simulink model "thermal_analysis"  (R2023b)
settings: Solver=VariableStepAuto  StartTime=0.0  StopTime=10.0  RelTol=1e-3
undefined symbols (not defined in the file): P_diode, P_mosfet, R_case_heatsink, R_heatsink_ambient, R_junction_case_diode, R_junction_case_mosfet, T_ambient
libraries: spsSeriesRLCBranchLib x6, spsControlledCurrentSourceLib x2, spsDCVoltageSourceLib x2, spsVoltageMeasurementLib x2, sps_lib x1
settings Model: Creator=ATAY  LastModifiedBy=ATAY

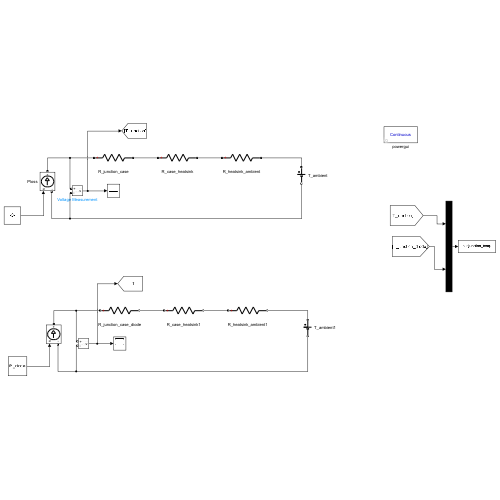
[thumbnail: Simulink's stored preview of the top-level diagram]
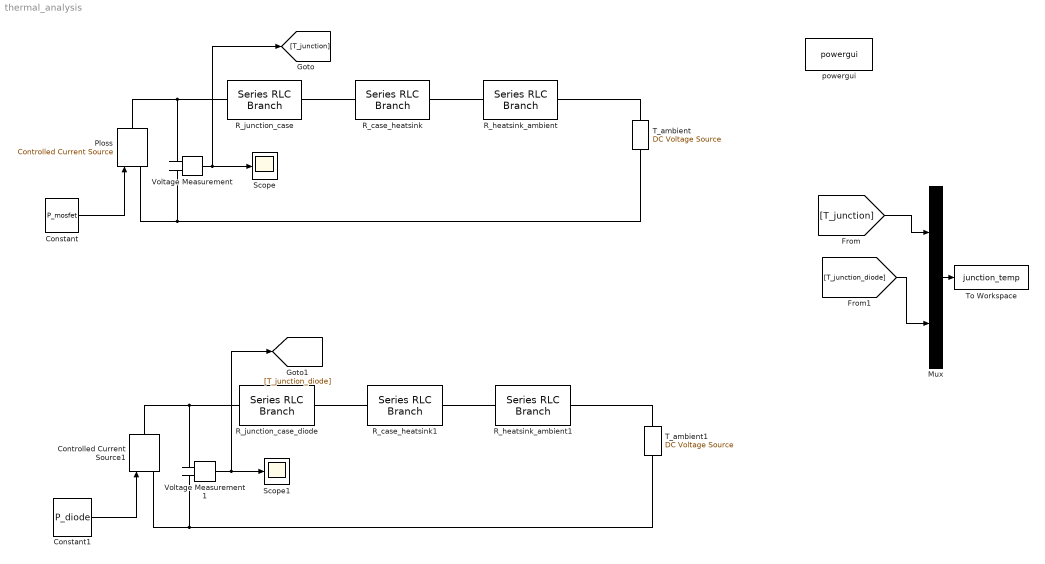
== system thermal_analysis ==
  Constant : Constant  Value=P_mosfet
  Constant1 : Constant  Value=P_diode
  Controlled Current Source1 : spsControlledCurrentSourceLib/Controlled Current Source  Initialize=on  Source_Type=DC  Amplitude=0  Phase=0  Frequency=0  Measurements=None
  Mux : Mux  Inputs=2
  Ploss : spsControlledCurrentSourceLib/Controlled Current Source  Initialize=on  Source_Type=DC  Amplitude=0  Phase=0  Frequency=0  Measurements=None
  R_case_heatsink : spsSeriesRLCBranchLib/Series RLC Branch  LConnTagsString=__new0  RConnTagsString=__new0  BranchType=R  Resistance=R_case_heatsink  Inductance=1e-3  SetiL0=off  InitialCurrent=0  Capacitance=1e-6  Setx0=off  InitialVoltage=0  Measurements=None
  R_case_heatsink1 : spsSeriesRLCBranchLib/Series RLC Branch  LConnTagsString=__new0  RConnTagsString=__new0  BranchType=R  Resistance=R_case_heatsink  Inductance=1e-3  SetiL0=off  InitialCurrent=0  Capacitance=1e-6  Setx0=off  InitialVoltage=0  Measurements=None
  R_heatsink_ambient : spsSeriesRLCBranchLib/Series RLC Branch  LConnTagsString=__new0  RConnTagsString=__new0  BranchType=R  Resistance=R_heatsink_ambient  Inductance=1e-3  SetiL0=off  InitialCurrent=0  Capacitance=1e-6  Setx0=off  InitialVoltage=0  Measurements=None
  R_heatsink_ambient1 : spsSeriesRLCBranchLib/Series RLC Branch  LConnTagsString=__new0  RConnTagsString=__new0  BranchType=R  Resistance=R_heatsink_ambient  Inductance=1e-3  SetiL0=off  InitialCurrent=0  Capacitance=1e-6  Setx0=off  InitialVoltage=0  Measurements=None
  R_junction_case : spsSeriesRLCBranchLib/Series RLC Branch  LConnTagsString=__new0  RConnTagsString=__new0  BranchType=R  Resistance=R_junction_case_mosfet  Inductance=1e-3  SetiL0=off  InitialCurrent=0  Capacitance=1e-6  Setx0=off  InitialVoltage=0  Measurements=None
  R_junction_case_diode : spsSeriesRLCBranchLib/Series RLC Branch  LConnTagsString=__new0  RConnTagsString=__new0  BranchType=R  Resistance=R_junction_case_diode  Inductance=1e-3  SetiL0=off  InitialCurrent=0  Capacitance=1e-6  Setx0=off  InitialVoltage=0  Measurements=None
  Scope : Scope
  Scope1 : Scope
  T_ambient : spsDCVoltageSourceLib/DC Voltage Source  Amplitude=T_ambient  Measurements=None
  T_ambient1 : spsDCVoltageSourceLib/DC Voltage Source  Amplitude=T_ambient  Measurements=None
  To Workspace : ToWorkspace  VariableName=junction_temp  SampleTime=-1
  Voltage Measurement : spsVoltageMeasurementLib/Voltage Measurement  PhasorSimulation=off  OutputType=Complex  PSBequivalent=0
  Voltage Measurement1 : spsVoltageMeasurementLib/Voltage Measurement  PhasorSimulation=off  OutputType=Complex  PSBequivalent=0
  powergui : sps_lib/powergui  Priority=1  SimulationMode=Continuous  SampleTime=50e-6  frequency=60  Iterations=50  frequencyindice=0  Pbase=100e6  ErrMax=1e-4  UnitsV=kV  UnitsW=MW  buscounter=0  FunctionMessages=off  echomessages=off  EnableUseOfTLC=off  CurrentSourceSwitches=off  DisableSnubberDevices=off  DisableRonSwitches=off  DisableVfSwitches=off  DisplayEquations=off  AutomaticDiscreteSolvers=off  SolverType=Tustin/Backward Euler (TBE)  Interpol=off  ExternalGateDelay=off  methode=off  Ts=100  x0status=blocks  SPID=on  SwTol=0  HookPort=off  NonlinearTolerance=1e-4  nMaxIteration=100  ContinueOnMaxIteration=off  RestoreLinks=warning  ResistiveCurrentMeasurement=off  Frange=[0:2:500]  Ylog=off  Xlog=on  ShowGrid=off  save=off  variable=ZData  structure=0  ZoomFFT=off  StartTime=0.0  cycles=1  DisplayStyle=1  fundamental=60  FreqAxis=off  MaxFrequency=1000  frequencyindicesteady=1  RmsSteady=1  display=off
  wires:
  Constant/1 -> Ploss/1
  Voltage Measurement/1 -> Scope/1, [T_junction]
  Voltage Measurement1/1 -> [T_junction_diode], Scope1/1
  Constant1/1 -> Controlled Current Source1/1
  Mux/1 -> To Workspace/1
  [T_junction_diode] -> Mux/2
  [T_junction] -> Mux/1
  connections:
  Ploss/RConn1 -- Voltage Measurement/LConn1 -- R_junction_case/LConn1
  R_case_heatsink/LConn1 -- R_junction_case/RConn1
  R_heatsink_ambient/LConn1 -- R_case_heatsink/RConn1
  T_ambient/RConn1 -- R_heatsink_ambient/RConn1
  T_ambient/LConn1 -- Voltage Measurement/LConn2 -- Ploss/LConn1
  Controlled Current Source1/RConn1 -- Voltage Measurement1/LConn1 -- R_junction_case_diode/LConn1
  T_ambient1/LConn1 -- Voltage Measurement1/LConn2 -- Controlled Current Source1/LConn1
  T_ambient1/RConn1 -- R_heatsink_ambient1/RConn1
  R_heatsink_ambient1/LConn1 -- R_case_heatsink1/RConn1
  R_case_heatsink1/LConn1 -- R_junction_case_diode/RConn1
